simulink model "Hospital_Context"  (R2025b)
settings: Solver=VariableStepAuto  StartTime=0.0  StopTime=10.0  RelTol=1e-3
settings Model: Creator=jakeo  LastModifiedBy=jakeo

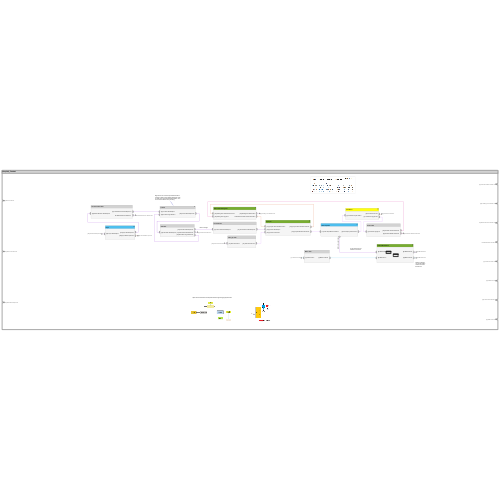
[thumbnail: Simulink's stored preview of the top-level diagram]
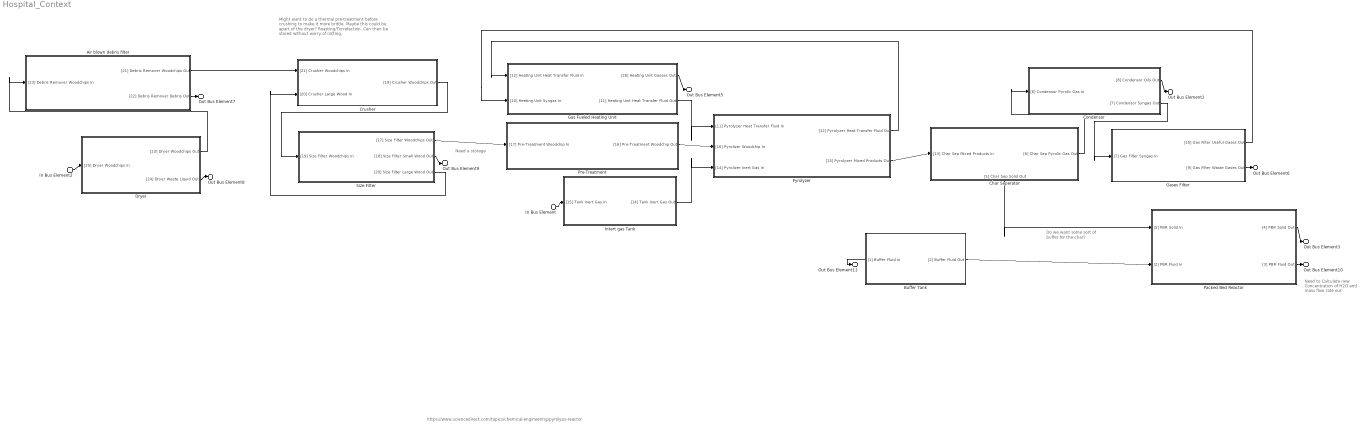
== system Hospital_Context ==
  note: Need a storage
  note: Might want to do a thermal pre-treatment before crushing to make it more brittle. Maybe this could be apart of the dryer? Roasting/Torrefaction. Can then be stored without worry of rotting.
  note: Need to Calculate new Concentration of H2O and mass flow rate out
  note: Do we want some sort of buffer for the char?
  note: https://www.sciencedirect.com/topics/chemical-engineering/pyrolysis-reactor
  In Bus Element2 : Inport  PortName=[25] World Woodchips Out
  In Bus Element : Inport  Port=2  PortName=[15] World Inert Gas Out
  Air blown debris filter : Subsystem
      settings: PortSchema="{\"entries\":[{\"content\":{\"headerSize\":26,\"margin\":15,\"minimumSpacing\":25,\"sides\":[{\"content\":{\"connectorIds\":[\"In1\"]},\"type\":\"ConnectorPlacement.EquallySpacedRectSide\",\"uuid\":\"cf9b5b84-c27e-443d-b9a2-3608ba31f5e4\"},{\"content\":{\"connectorIds\":[\"Out1\",\"Out2\"],\"side\":\"RIGHT\"},\"type\":\"ConnectorPlacement.EquallySpacedRectSide\",\"uuid\":\"efa89936-2b13-4422-9975-be719059dbdc\"},{\"content\":{\"side\":\"TOP\"},\"type\":\"ConnectorPlacement.EquallySpacedRectSide\",\"uuid\":\"249a79e9-4422-4697-8fba-0436c9decabf\"},{\"content\":{\"side\":\"BOTTOM\"},\"type\":\"ConnectorPlacement.EquallySpacedRectSide\",\"uuid\":\"86a2852a-f48b-482a-862b-0840c2ecc386\"}]},\"type\":\"ConnectorPlacement.EquallySpacedConnector\",\"uuid\":\"9d78504a-b513-4a9b-89b2-eac19dc7bc23\"}],\"packageUris\":[\"http://schema.mathworks.com/mf0/Connector/R2020b\"],\"version\":\"1.0\"}"
  Buffer Tank : Subsystem
      settings: PortSchema="{\"entries\":[{\"content\":{\"headerSize\":26,\"margin\":15,\"minimumSpacing\":25,\"sides\":[{\"content\":{\"connectorIds\":[\"Out1\"]},\"type\":\"ConnectorPlacement.EquallySpacedRectSide\",\"uuid\":\"cf9b5b84-c27e-443d-b9a2-3608ba31f5e4\"},{\"content\":{\"connectorIds\":[\"Out2\"],\"side\":\"RIGHT\"},\"type\":\"ConnectorPlacement.EquallySpacedRectSide\",\"uuid\":\"efa89936-2b13-4422-9975-be719059dbdc\"},{\"content\":{\"side\":\"TOP\"},\"type\":\"ConnectorPlacement.EquallySpacedRectSide\",\"uuid\":\"249a79e9-4422-4697-8fba-0436c9decabf\"}]},\"type\":\"ConnectorPlacement.EquallySpacedConnector\",\"uuid\":\"9d78504a-b513-4a9b-89b2-eac19dc7bc23\"}],\"packageUris\":[\"http://schema.mathworks.com/mf0/Connector/R2020b\"],\"version\":\"1.0\"}"
  Char Seperator : Subsystem
      settings: PortSchema="{\"entries\":[{\"content\":{\"headerSize\":26,\"margin\":15,\"minimumSpacing\":25,\"sides\":[{\"content\":{\"connectorIds\":[\"In1\"]},\"type\":\"ConnectorPlacement.EquallySpacedRectSide\",\"uuid\":\"fa1dbd3d-b57d-47b9-b4ef-0fe90e72294f\"},{\"content\":{\"connectorIds\":[\"Out1\"],\"side\":\"RIGHT\"},\"type\":\"ConnectorPlacement.EquallySpacedRectSide\",\"uuid\":\"948d51fa-2dfa-4f43-89d3-5e64c8759b0a\"},{\"content\":{\"side\":\"TOP\"},\"type\":\"ConnectorPlacement.EquallySpacedRectSide\",\"uuid\":\"ae7cb2a6-ad1d-4ea0-b46a-3d468529a90e\"},{\"content\":{\"connectorIds\":[\"Out2\"],\"side\":\"BOTTOM\"},\"type\":\"ConnectorPlacement.EquallySpacedRectSide\",\"uuid\":\"a440eaf4-fb0e-4071-9eb7-73669642cd6c\"}]},\"type\":\"ConnectorPlacement.EquallySpacedConnector\",\"uuid\":\"9e4666f3-ab23-41a5-b5e5-84e2e52e58ec\"}],\"packageUris\":[\"http://schema.mathworks.com/mf0/Connector/R2020b\"],\"version\":\"1.0\"}"
  Condensor : Subsystem
      settings: PortSchema="{\"entries\":[{\"content\":{\"headerSize\":26,\"margin\":15,\"minimumSpacing\":25,\"sides\":[{\"content\":{\"connectorIds\":[\"In1\"]},\"type\":\"ConnectorPlacement.EquallySpacedRectSide\",\"uuid\":\"fa1dbd3d-b57d-47b9-b4ef-0fe90e72294f\"},{\"content\":{\"connectorIds\":[\"Out2\",\"Out1\"],\"side\":\"RIGHT\"},\"type\":\"ConnectorPlacement.EquallySpacedRectSide\",\"uuid\":\"948d51fa-2dfa-4f43-89d3-5e64c8759b0a\"},{\"content\":{\"side\":\"TOP\"},\"type\":\"ConnectorPlacement.EquallySpacedRectSide\",\"uuid\":\"ae7cb2a6-ad1d-4ea0-b46a-3d468529a90e\"}]},\"type\":\"ConnectorPlacement.EquallySpacedConnector\",\"uuid\":\"9e4666f3-ab23-41a5-b5e5-84e2e52e58ec\"}],\"packageUris\":[\"http://schema.mathworks.com/mf0/Connector/R2020b\"],\"version\":\"1.0\"}"
  Crusher : Subsystem
      settings: PortSchema="{\"entries\":[{\"content\":{\"headerSize\":26,\"margin\":15,\"minimumSpacing\":25,\"sides\":[{\"content\":{\"connectorIds\":[\"In2\",\"In1\"]},\"type\":\"ConnectorPlacement.EquallySpacedRectSide\",\"uuid\":\"fa1dbd3d-b57d-47b9-b4ef-0fe90e72294f\"},{\"content\":{\"connectorIds\":[\"Out1\"],\"side\":\"RIGHT\"},\"type\":\"ConnectorPlacement.EquallySpacedRectSide\",\"uuid\":\"948d51fa-2dfa-4f43-89d3-5e64c8759b0a\"},{\"content\":{\"side\":\"TOP\"},\"type\":\"ConnectorPlacement.EquallySpacedRectSide\",\"uuid\":\"ae7cb2a6-ad1d-4ea0-b46a-3d468529a90e\"}]},\"type\":\"ConnectorPlacement.EquallySpacedConnector\",\"uuid\":\"9e4666f3-ab23-41a5-b5e5-84e2e52e58ec\"}],\"packageUris\":[\"http://schema.mathworks.com/mf0/Connector/R2020b\"],\"version\":\"1.0\"}"
  Dryer : Subsystem
      settings: PortSchema="{\"entries\":[{\"content\":{\"headerSize\":26,\"margin\":15,\"minimumSpacing\":25,\"sides\":[{\"content\":{\"connectorIds\":[\"In1\"]},\"type\":\"ConnectorPlacement.EquallySpacedRectSide\",\"uuid\":\"fa1dbd3d-b57d-47b9-b4ef-0fe90e72294f\"},{\"content\":{\"connectorIds\":[\"Out1\",\"Out2\"],\"side\":\"RIGHT\"},\"type\":\"ConnectorPlacement.EquallySpacedRectSide\",\"uuid\":\"948d51fa-2dfa-4f43-89d3-5e64c8759b0a\"},{\"content\":{\"side\":\"TOP\"},\"type\":\"ConnectorPlacement.EquallySpacedRectSide\",\"uuid\":\"ae7cb2a6-ad1d-4ea0-b46a-3d468529a90e\"}]},\"type\":\"ConnectorPlacement.EquallySpacedConnector\",\"uuid\":\"9e4666f3-ab23-41a5-b5e5-84e2e52e58ec\"}],\"packageUris\":[\"http://schema.mathworks.com/mf0/Connector/R2020b\"],\"version\":\"1.0\"}"
  Gas Fueled Heating Unit : Subsystem
      settings: PortSchema="{\"entries\":[{\"content\":{\"headerSize\":26,\"margin\":15,\"minimumSpacing\":25,\"sides\":[{\"content\":{\"connectorIds\":[\"In2\",\"In1\"]},\"type\":\"ConnectorPlacement.EquallySpacedRectSide\",\"uuid\":\"fa1dbd3d-b57d-47b9-b4ef-0fe90e72294f\"},{\"content\":{\"connectorIds\":[\"Out2\",\"Out1\"],\"side\":\"RIGHT\"},\"type\":\"ConnectorPlacement.EquallySpacedRectSide\",\"uuid\":\"948d51fa-2dfa-4f43-89d3-5e64c8759b0a\"},{\"content\":{\"side\":\"TOP\"},\"type\":\"ConnectorPlacement.EquallySpacedRectSide\",\"uuid\":\"ae7cb2a6-ad1d-4ea0-b46a-3d468529a90e\"}]},\"type\":\"ConnectorPlacement.EquallySpacedConnector\",\"uuid\":\"9e4666f3-ab23-41a5-b5e5-84e2e52e58ec\"}],\"packageUris\":[\"http://schema.mathworks.com/mf0/Connector/R2020b\"],\"version\":\"1.0\"}"
  Gases Filter : Subsystem
      settings: PortSchema="{\"entries\":[{\"content\":{\"headerSize\":26,\"margin\":15,\"minimumSpacing\":25,\"sides\":[{\"content\":{\"connectorIds\":[\"In1\"]},\"type\":\"ConnectorPlacement.EquallySpacedRectSide\",\"uuid\":\"cf9b5b84-c27e-443d-b9a2-3608ba31f5e4\"},{\"content\":{\"connectorIds\":[\"Out1\",\"Out2\"],\"side\":\"RIGHT\"},\"type\":\"ConnectorPlacement.EquallySpacedRectSide\",\"uuid\":\"efa89936-2b13-4422-9975-be719059dbdc\"},{\"content\":{\"side\":\"TOP\"},\"type\":\"ConnectorPlacement.EquallySpacedRectSide\",\"uuid\":\"249a79e9-4422-4697-8fba-0436c9decabf\"}]},\"type\":\"ConnectorPlacement.EquallySpacedConnector\",\"uuid\":\"9d78504a-b513-4a9b-89b2-eac19dc7bc23\"}],\"packageUris\":[\"http://schema.mathworks.com/mf0/Connector/R2020b\"],\"version\":\"1.0\"}"
  Intert gas Tank : Subsystem
      settings: PortSchema="{\"entries\":[{\"content\":{\"headerSize\":26,\"margin\":15,\"minimumSpacing\":25,\"sides\":[{\"content\":{\"connectorIds\":[\"In1\"]},\"type\":\"ConnectorPlacement.EquallySpacedRectSide\",\"uuid\":\"cf9b5b84-c27e-443d-b9a2-3608ba31f5e4\"},{\"content\":{\"connectorIds\":[\"Out1\"],\"side\":\"RIGHT\"},\"type\":\"ConnectorPlacement.EquallySpacedRectSide\",\"uuid\":\"efa89936-2b13-4422-9975-be719059dbdc\"},{\"content\":{\"side\":\"TOP\"},\"type\":\"ConnectorPlacement.EquallySpacedRectSide\",\"uuid\":\"249a79e9-4422-4697-8fba-0436c9decabf\"}]},\"type\":\"ConnectorPlacement.EquallySpacedConnector\",\"uuid\":\"9d78504a-b513-4a9b-89b2-eac19dc7bc23\"}],\"packageUris\":[\"http://schema.mathworks.com/mf0/Connector/R2020b\"],\"version\":\"1.0\"}"
  Packed Bed Reactor : Subsystem
      settings: PortSchema="{\"entries\":[{\"content\":{\"headerSize\":26,\"margin\":15,\"minimumSpacing\":25,\"sides\":[{\"content\":{\"connectorIds\":[\"In1\",\"In2\"]},\"type\":\"ConnectorPlacement.EquallySpacedRectSide\",\"uuid\":\"fa1dbd3d-b57d-47b9-b4ef-0fe90e72294f\"},{\"content\":{\"connectorIds\":[\"Out2\",\"Out1\"],\"side\":\"RIGHT\"},\"type\":\"ConnectorPlacement.EquallySpacedRectSide\",\"uuid\":\"948d51fa-2dfa-4f43-89d3-5e64c8759b0a\"},{\"content\":{\"side\":\"TOP\"},\"type\":\"ConnectorPlacement.EquallySpacedRectSide\",\"uuid\":\"ae7cb2a6-ad1d-4ea0-b46a-3d468529a90e\"},{\"content\":{\"side\":\"BOTTOM\"},\"type\":\"ConnectorPlacement.EquallySpacedRectSide\",\"uuid\":\"dc29dfe4-3980-46f5-bd0d-b60b93a30b71\"}]},\"type\":\"ConnectorPlacement.EquallySpacedConnector\",\"uuid\":\"9e4666f3-ab23-41a5-b5e5-84e2e52e58ec\"}],\"packageUris\":[\"http://schema.mathworks.com/mf0/Connector/R2020b\"],\"version\":\"1.0\"}"
  Pre-Treatment : Subsystem
      settings: PortSchema="{\"entries\":[{\"content\":{\"headerSize\":26,\"margin\":15,\"minimumSpacing\":25,\"sides\":[{\"content\":{\"connectorIds\":[\"In1\"]},\"type\":\"ConnectorPlacement.EquallySpacedRectSide\",\"uuid\":\"cf9b5b84-c27e-443d-b9a2-3608ba31f5e4\"},{\"content\":{\"connectorIds\":[\"Out1\"],\"side\":\"RIGHT\"},\"type\":\"ConnectorPlacement.EquallySpacedRectSide\",\"uuid\":\"efa89936-2b13-4422-9975-be719059dbdc\"},{\"content\":{\"side\":\"TOP\"},\"type\":\"ConnectorPlacement.EquallySpacedRectSide\",\"uuid\":\"249a79e9-4422-4697-8fba-0436c9decabf\"}]},\"type\":\"ConnectorPlacement.EquallySpacedConnector\",\"uuid\":\"9d78504a-b513-4a9b-89b2-eac19dc7bc23\"}],\"packageUris\":[\"http://schema.mathworks.com/mf0/Connector/R2020b\"],\"version\":\"1.0\"}"
  Pyrolyzer : Subsystem
      settings: PortSchema="{\"entries\":[{\"content\":{\"headerSize\":26,\"margin\":15,\"minimumSpacing\":25,\"sides\":[{\"content\":{\"connectorIds\":[\"In3\",\"In1\",\"In2\"]},\"type\":\"ConnectorPlacement.EquallySpacedRectSide\",\"uuid\":\"fa1dbd3d-b57d-47b9-b4ef-0fe90e72294f\"},{\"content\":{\"connectorIds\":[\"Out1\",\"Out2\"],\"side\":\"RIGHT\"},\"type\":\"ConnectorPlacement.EquallySpacedRectSide\",\"uuid\":\"948d51fa-2dfa-4f43-89d3-5e64c8759b0a\"},{\"content\":{\"side\":\"TOP\"},\"type\":\"ConnectorPlacement.EquallySpacedRectSide\",\"uuid\":\"ae7cb2a6-ad1d-4ea0-b46a-3d468529a90e\"},{\"content\":{\"side\":\"BOTTOM\"},\"type\":\"ConnectorPlacement.EquallySpacedRectSide\",\"uuid\":\"c41ca62f-2536-4c7c-93b5-233085d0098c\"}]},\"type\":\"ConnectorPlacement.EquallySpacedConnector\",\"uuid\":\"9e4666f3-ab23-41a5-b5e5-84e2e52e58ec\"}],\"packageUris\":[\"http://schema.mathworks.com/mf0/Connector/R2020b\"],\"version\":\"1.0\"}"
  Size Filter : Subsystem
      settings: PortSchema="{\"entries\":[{\"content\":{\"headerSize\":26,\"margin\":15,\"minimumSpacing\":25,\"sides\":[{\"content\":{\"connectorIds\":[\"In1\"]},\"type\":\"ConnectorPlacement.EquallySpacedRectSide\",\"uuid\":\"cf9b5b84-c27e-443d-b9a2-3608ba31f5e4\"},{\"content\":{\"connectorIds\":[\"Out2\",\"Out3\",\"Out1\"],\"side\":\"RIGHT\"},\"type\":\"ConnectorPlacement.EquallySpacedRectSide\",\"uuid\":\"efa89936-2b13-4422-9975-be719059dbdc\"},{\"content\":{\"side\":\"TOP\"},\"type\":\"ConnectorPlacement.EquallySpacedRectSide\",\"uuid\":\"249a79e9-4422-4697-8fba-0436c9decabf\"}]},\"type\":\"ConnectorPlacement.EquallySpacedConnector\",\"uuid\":\"9d78504a-b513-4a9b-89b2-eac19dc7bc23\"}],\"packageUris\":[\"http://schema.mathworks.com/mf0/Connector/R2020b\"],\"version\":\"1.0\"}"
  Out Bus Element6 : Outport  PortName=[9] Gas Filter Waste Gases Out
  Out Bus Element5 : Outport  Port=2  PortName=[26] Heating Unit Gasses Out
  Out Bus Element7 : Outport  Port=3  PortName=[22] Debris Remover Debris Out
  Out Bus Element8 : Outport  Port=4  PortName=[24] World Waste Liquid In
  Out Bus Element2 : Outport  Port=5  PortName=[8] Condensor Oils Out
  Out Bus Element10 : Outport  Port=6  PortName=[3] PBR Fluid Out
  Out Bus Element11 : Outport  Port=7  PortName=[1] World Fluid Out
  Out Bus Element9 : Outport  Port=8  PortName=[18] World Small Wood In
  Out Bus Element3 : Outport  Port=9  PortName=[4] PBR Solid Out
  wires:
  Pyrolyzer/2("[13] Pyrolyzer Mixed Products Out") -> Char Seperator/1("[13] Char Sep Mixed Products In")
  Packed Bed Reactor/2("[4] PBR Solid Out") -> Out Bus Element3/1
  Packed Bed Reactor/1("[3] PBR Fluid Out") -> Out Bus Element10/1
  Buffer Tank/2("[2] Buffer Fluid Out") -> Packed Bed Reactor/2("[2] PBR Fluid In")
  In Bus Element2/1 -> Dryer/1("[25] Dryer Woodchips In")
  Dryer/1("[23] Dryer Woodchips Out") -> Air blown debris filter/1("[23] Debris Remover Woodchips In")
  Crusher/1("[19] Crusher Woodchips Out") -> Size Filter/1("[19] Size Filter Woodchips In")
  Gas Fueled Heating Unit/1("[11] Heating Unit Heat Transfer Fluid Out") -> Pyrolyzer/3("[11] Pyrolyzer Heat Transfer Fluid In")
  Char Seperator/2("[5] Char Sep Solid Out") -> Packed Bed Reactor/1("[5] PBR Solid In")
  Dryer/2("[24] Dryer Waste Liquid Out") -> Out Bus Element8/1
  Char Seperator/1("[6] Char Sep Pyrolic Gas Out") -> Condensor/1("[6] Condensor Pyrolic Gas In")
  Condensor/2("[8] Condensor Oils Out") -> Out Bus Element2/1
  Air blown debris filter/1("[21] Debris Remover Woodchips Out") -> Crusher/2("[21] Crusher Woodchips In")
  Pyrolyzer/1("[12] Pyrolyzer Heat Transfer Fluid Out") -> Gas Fueled Heating Unit/2("[12] Heating Unit Heat Transfer Fluid In")
  Size Filter/2("[17] Size Filter Woodchips Out") -> Pre-Treatment/1("[17] Pre-Treatment Woodchip In")
  Pre-Treatment/1("[16] Pre-Treatment Woodchip Out") -> Pyrolyzer/1("[16] Pyrolizer Woodchip In")
  Size Filter/1("[20] Size Filter Large Wood Out") -> Crusher/1("[20] Crusher Large Wood In")
  Size Filter/3("[18] Size Filter Small Wood Out") -> Out Bus Element9/1
  Gas Fueled Heating Unit/2("[26] Heating Unit Gasses Out") -> Out Bus Element5/1
  Condensor/1("[7] Condensor Syngas Out") -> Gases Filter/1("[7] Gas Filter Syngas In")
  Gases Filter/2("[9] Gas Filter Waste Gases Out") -> Out Bus Element6/1
  Gases Filter/1("[10] Gas Filter Useful Gases Out") -> Gas Fueled Heating Unit/1("[10] Heating Unit Syngas In")
  Air blown debris filter/2("[22] Debris Remover Debris Out") -> Out Bus Element7/1
  Intert gas Tank/1("[14] Tank Inert Gas Out") -> Pyrolyzer/2("[14] Pyrolizer Inert Gas In")
  Buffer Tank/1("[1] Buffer Fluid In") -> Out Bus Element11/1
  In Bus Element/1 -> Intert gas Tank/1("[15] Tank Inert Gas In")

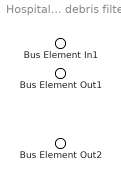
== system Hospital_Context/Air blown debris filter ==
  Bus Element In1 : Inport  PortName=[23] Debris Remover Woodchips In
  Bus Element Out1 : Outport  PortName=[21] Debris Remover Woodchips Out
  Bus Element Out2 : Outport  Port=2  PortName=[22] Debris Remover Debris Out

== system Hospital_Context/Buffer Tank ==
  Bus Element Out2 : Outport  PortName=[1] Buffer Fluid In
  Bus Element Out1 : Outport  Port=2  PortName=[2] Buffer Fluid Out

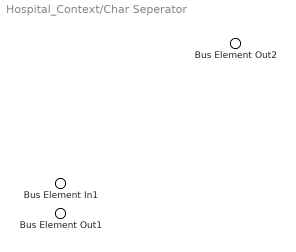
== system Hospital_Context/Char Seperator ==
  Bus Element In1 : Inport  PortName=[13] Char Sep Mixed Products In
  Bus Element Out2 : Outport  PortName=[6] Char Sep Pyrolic Gas Out
  Bus Element Out1 : Outport  Port=2  PortName=[5] Char Sep Solid Out

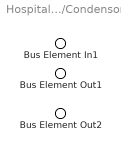
== system Hospital_Context/Condensor ==
  Bus Element In1 : Inport  PortName=[6] Condensor Pyrolic Gas In
  Bus Element Out1 : Outport  PortName=[7] Condensor Syngas Out
  Bus Element Out2 : Outport  Port=2  PortName=[8] Condensor Oils Out

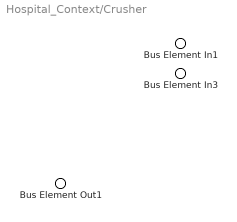
== system Hospital_Context/Crusher ==
  Bus Element In3 : Inport  PortName=[20] Crusher Large Wood In
  Bus Element In1 : Inport  Port=2  PortName=[21] Crusher Woodchips In
  Bus Element Out1 : Outport  PortName=[19] Crusher Woodchips Out

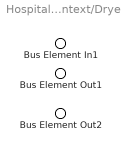
== system Hospital_Context/Dryer ==
  Bus Element In1 : Inport  PortName=[25] Dryer Woodchips In
  Bus Element Out1 : Outport  PortName=[23] Dryer Woodchips Out
  Bus Element Out2 : Outport  Port=2  PortName=[24] Dryer Waste Liquid Out

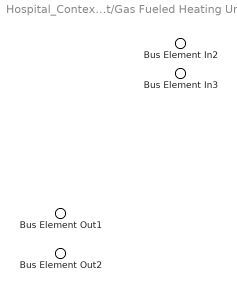
== system Hospital_Context/Gas Fueled Heating Unit ==
  Bus Element In3 : Inport  PortName=[10] Heating Unit Syngas In
  Bus Element In2 : Inport  Port=2  PortName=[12] Heating Unit Heat Transfer Fluid In
  Bus Element Out1 : Outport  PortName=[11] Heating Unit Heat Transfer Fluid Out
  Bus Element Out2 : Outport  Port=2  PortName=[26] Heating Unit Gasses Out

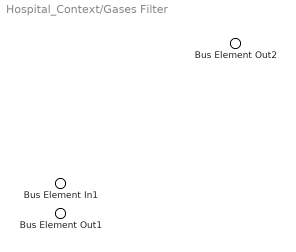
== system Hospital_Context/Gases Filter ==
  Bus Element In1 : Inport  PortName=[7] Gas Filter Syngas In
  Bus Element Out2 : Outport  PortName=[10] Gas Filter Useful Gases Out
  Bus Element Out1 : Outport  Port=2  PortName=[9] Gas Filter Waste Gases Out

== system Hospital_Context/Intert gas Tank ==
  Bus Element In1 : Inport  PortName=[15] Tank Inert Gas In
  Bus Element Out1 : Outport  PortName=[14] Tank Inert Gas Out

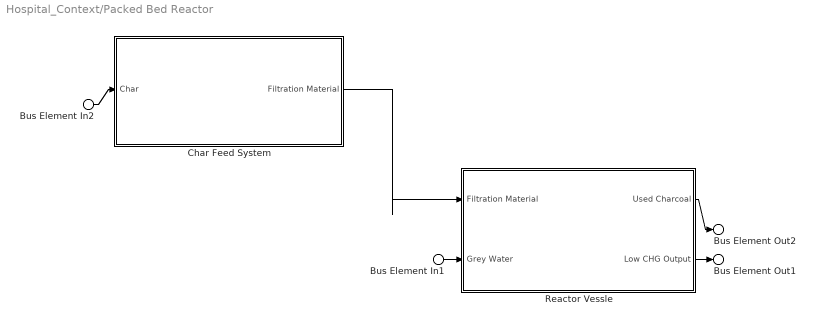
== system Hospital_Context/Packed Bed Reactor ==
  Bus Element In2 : Inport  PortName=[5] PBR Solid In
  Bus Element In1 : Inport  Port=2  PortName=[2] PBR Fluid In
  Char Feed System : Subsystem
      settings: PortSchema="{\"entries\":[{\"content\":{\"headerSize\":26,\"margin\":15,\"minimumSpacing\":25,\"sides\":[{\"content\":{\"connectorIds\":[\"In1\"]},\"type\":\"ConnectorPlacement.EquallySpacedRectSide\",\"uuid\":\"fa1dbd3d-b57d-47b9-b4ef-0fe90e72294f\"},{\"content\":{\"connectorIds\":[\"Out1\"],\"side\":\"RIGHT\"},\"type\":\"ConnectorPlacement.EquallySpacedRectSide\",\"uuid\":\"948d51fa-2dfa-4f43-89d3-5e64c8759b0a\"},{\"content\":{\"side\":\"TOP\"},\"type\":\"ConnectorPlacement.EquallySpacedRectSide\",\"uuid\":\"ae7cb2a6-ad1d-4ea0-b46a-3d468529a90e\"}]},\"type\":\"ConnectorPlacement.EquallySpacedConnector\",\"uuid\":\"9e4666f3-ab23-41a5-b5e5-84e2e52e58ec\"}],\"packageUris\":[\"http://schema.mathworks.com/mf0/Connector/R2020b\"],\"version\":\"1.0\"}"
  Reactor Vessle : Subsystem
      settings: PortSchema="{\"entries\":[{\"content\":{\"headerSize\":26,\"margin\":15,\"minimumSpacing\":25,\"sides\":[{\"content\":{\"connectorIds\":[\"In1\",\"In2\"]},\"type\":\"ConnectorPlacement.EquallySpacedRectSide\",\"uuid\":\"fa1dbd3d-b57d-47b9-b4ef-0fe90e72294f\"},{\"content\":{\"connectorIds\":[\"Out1\",\"Out2\"],\"side\":\"RIGHT\"},\"type\":\"ConnectorPlacement.EquallySpacedRectSide\",\"uuid\":\"948d51fa-2dfa-4f43-89d3-5e64c8759b0a\"},{\"content\":{\"side\":\"TOP\"},\"type\":\"ConnectorPlacement.EquallySpacedRectSide\",\"uuid\":\"ae7cb2a6-ad1d-4ea0-b46a-3d468529a90e\"}]},\"type\":\"ConnectorPlacement.EquallySpacedConnector\",\"uuid\":\"9e4666f3-ab23-41a5-b5e5-84e2e52e58ec\"}],\"packageUris\":[\"http://schema.mathworks.com/mf0/Connector/R2020b\"],\"version\":\"1.0\"}"
  Bus Element Out1 : Outport  PortName=[3] PBR Fluid Out
  Bus Element Out2 : Outport  Port=2  PortName=[4] PBR Solid Out
  wires:
  Bus Element In1/1 -> Reactor Vessle/2(Grey Water)
  Char Feed System/1(Filtration Material) -> Reactor Vessle/1(Filtration Material)
  Reactor Vessle/1(Used Charcoal) -> Bus Element Out2/1
  Reactor Vessle/2(Low CHG Output) -> Bus Element Out1/1
  Bus Element In2/1 -> Char Feed System/1(Char)

== system Hospital_Context/Pre-Treatment ==
  Bus Element In1 : Inport  PortName=[17] Pre-Treatment Woodchip In
  Bus Element Out1 : Outport  PortName=[16] Pre-Treatment Woodchip Out

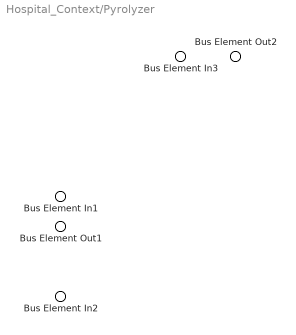
== system Hospital_Context/Pyrolyzer ==
  Bus Element In1 : Inport  PortName=[16] Pyrolizer Woodchip In
  Bus Element In3 : Inport  Port=2  PortName=[14] Pyrolizer Inert Gas In
  Bus Element In2 : Inport  Port=3  PortName=[11] Pyrolyzer Heat Transfer Fluid In
  Bus Element Out2 : Outport  PortName=[12] Pyrolyzer Heat Transfer Fluid Out
  Bus Element Out1 : Outport  Port=2  PortName=[13] Pyrolyzer Mixed Products Out

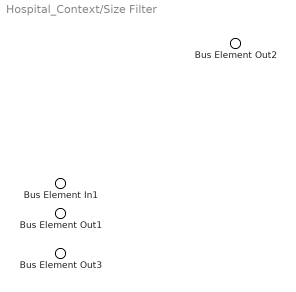
== system Hospital_Context/Size Filter ==
  Bus Element In1 : Inport  PortName=[19] Size Filter Woodchips In
  Bus Element Out2 : Outport  PortName=[20] Size Filter Large Wood Out
  Bus Element Out1 : Outport  Port=2  PortName=[17] Size Filter Woodchips Out
  Bus Element Out3 : Outport  Port=3  PortName=[18] Size Filter Small Wood Out

== system Hospital_Context/Packed Bed Reactor/Char Feed System ==
  Bus Element In1 : Inport  PortName=Char
  Bus Element Out1 : Outport  PortName=Filtration Material

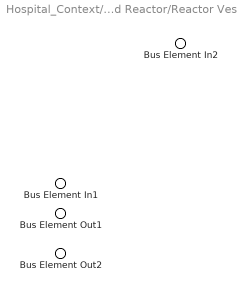
== system Hospital_Context/Packed Bed Reactor/Reactor Vessle ==
  Bus Element In2 : Inport  PortName=Filtration Material
  Bus Element In1 : Inport  Port=2  PortName=Grey Water
  Bus Element Out1 : Outport  PortName=Used Charcoal
  Bus Element Out2 : Outport  Port=2  PortName=Low CHG Output
